simulink library "m3_common_lib"  (R2021b)
settings: Solver=ode45  StartTime=0.0  StopTime=10.0  RelTol=1e-3
undefined symbols (not defined in the file or in its folder): ACCEL_PRE_MULT, APDT_SrvcMgr_IRVHVDCSubFcnReq, C_C1GearNumbers, C_C1GearRatios, C_Calibration, C_DitherWaveform, C_GearOffset, C_GearRatioIn, C_GearRatioInverseOut, C_GearRatioOut, CLUTCH_INNER_LOOP_UPDATE_RATE, CONSTANT, DEGRADED_MODE_SIZE, Dem_EventStatusType, DiscIntNeverNeededParam, F_FAULT_ENUM, F_NOFAULT, F_OUTOFRANGE, F_RATELIMIT, FALSE, FMI14_SPECIAL_INSTRUCTIONS, FMI20_DATA_DRIFTED_HIGH, FMI21_DATA_DRIFTED_LOW, FMI29_RESERVED_FOR_SAE_ASSIGNMENT, FMI30_RESERVED_FOR_SAE_ASSIGNMENT, FMI31_CONDITION_EXISTS, FMI32_NO_FAULT, IC, k_accel, k_mean, MAX_UINT32, MEAN_PRE_MULT, NTriggers, QLTY_SIGNAL_FAILED, QLTY_SIGNAL_FULLY_FUNCTION, QLTY_SIGNAL_SUBSTITUTED_BY_1ST_CHOICE, QLTY_SIGNAL_SUBSTITUTED_BY_2ND_CHOICE, QLTY_SIGNAL_SUBSTITUTED_BY_3RD_CHOICE, QLTY_SIGNAL_SUBSTITUTED_BY_4TH_CHOICE, SAMPLE_TIME_100us, simin, T_TestPoint, TF_FALSE, TF_TRUE, TimeStep, TRUE, WORKSPACE_UPDATE_RATE, Zero, ZERO
libraries: $bdroot x121, simulink x23, simulink_extras x4, MBD_EPS_Local_Blockset x4
(part 6 of 10)

== system m3_common_lib/Diagnostics/OOR Fault Detect Enum ==
  note: Common Library::Diagnostics::Out of Range Fault Detection with Enable for Enum
  in : Inport
  Enable : Inport  Port=2
  Logical Operator1 : Logic  Operator=NOT  AllPortsSameDT=off
  Switch : Switch  Criteria=u2 ~= 0
  detect fault : Subsystem
  false : Constant  Value=false  OutDataTypeStr=boolean
  out : Outport  VectorParamsAs1DForOutWhenUnconnected=off
  fault? : Outport  Port=2  VectorParamsAs1DForOutWhenUnconnected=off
  wires:
  Enable/1 -> detect fault/Enable, Logical Operator1/1
  Switch/1 -> fault?/1
  false/1 -> Switch/1
  detect fault/1(fault set) -> Switch/3
  in/1 -> detect fault/1(In1), out/1
  Logical Operator1/1 -> Switch/2

== system m3_common_lib/Diagnostics/OOR Fault Detection ==
  note: Common Library::Diagnostics::Out of Range Fault Detection with Enable
  in : Inport
  Enable : Inport  Port=2
  Logical Operator1 : Logic  Operator=OR  AllPortsSameDT=off
  Logical Operator2 : Logic  Operator=NOT  AllPortsSameDT=off
  Logical Operator3 : Logic  Operator=NOT  AllPortsSameDT=off
  Logical Operator4 : Logic  Operator=NOT  AllPortsSameDT=off
  Switch : Switch  Criteria=u2 ~= 0
  applyLimits : Constant  Value=applyLimits
  detect fault : Subsystem
  false : Constant  Value=false  OutDataTypeStr=boolean
  out : Outport  VectorParamsAs1DForOutWhenUnconnected=off
  fault? : Outport  Port=2  VectorParamsAs1DForOutWhenUnconnected=off
  wires:
  Enable/1 -> Logical Operator3/1
  in/1 -> out/1, detect fault/1(In1)
  applyLimits/1 -> Logical Operator2/1
  Logical Operator1/1 -> Switch/2, Logical Operator4/1
  detect fault/1(fault set) -> Switch/3
  false/1 -> Switch/1
  Switch/1 -> fault?/1
  Logical Operator2/1 -> Logical Operator1/1
  Logical Operator3/1 -> Logical Operator1/2
  Logical Operator4/1 -> detect fault/Enable

== system m3_common_lib/Diagnostics/SetFMI ==
  FMI_in : Inport  OutDataTypeStr=uint8  PortDimensions=1
  Active1 : Inport  Port=2  OutDataTypeStr=boolean  PortDimensions=1
  Active2 : Inport  Port=3  OutDataTypeStr=boolean  PortDimensions=1
  Active3 : Inport  Port=4  OutDataTypeStr=boolean  PortDimensions=1
  Active4 : Inport  Port=5  OutDataTypeStr=boolean  PortDimensions=1
  Active5 : Inport  Port=6  OutDataTypeStr=boolean  PortDimensions=1
  Active6 : Inport  Port=7  OutDataTypeStr=boolean  PortDimensions=1
  Active7 : Inport  Port=8  OutDataTypeStr=boolean  PortDimensions=1
  Constant : Constant  Value=PRIORITY_1_FMI
  Constant1 : Constant  Value=PRIORITY_2_FMI
  Constant2 : Constant  Value=PRIORITY_3_FMI
  Constant3 : Constant  Value=PRIORITY_4_FMI
  Constant4 : Constant  Value=PRIORITY_5_FMI
  Constant5 : Constant  Value=PRIORITY_6_FMI
  Constant6 : Constant  Value=PRIORITY_7_FMI
  IF_ELSE_LADDER : Subsystem  TreatAsAtomicUnit=on
      settings: RTWSystemCode=Inline
  FMI_out : Outport  VectorParamsAs1DForOutWhenUnconnected=off
  wires:
  IF_ELSE_LADDER/1(FMI_out) -> FMI_out/1
  Active7/1 -> IF_ELSE_LADDER/8(Active7)
  Active6/1 -> IF_ELSE_LADDER/7(Active6)
  Active5/1 -> IF_ELSE_LADDER/6(Active5)
  Active4/1 -> IF_ELSE_LADDER/5(Active4)
  Active3/1 -> IF_ELSE_LADDER/4(Active3)
  Active2/1 -> IF_ELSE_LADDER/3(Active2)
  Active1/1 -> IF_ELSE_LADDER/2(Active1)
  FMI_in/1 -> IF_ELSE_LADDER/1(FMI_in)
  Constant6/1 -> IF_ELSE_LADDER/15(FMI_7)
  Constant5/1 -> IF_ELSE_LADDER/14(FMI_6)
  Constant4/1 -> IF_ELSE_LADDER/13(FMI_5)
  Constant3/1 -> IF_ELSE_LADDER/12(FMI_4)
  Constant2/1 -> IF_ELSE_LADDER/11(FMI_3)
  Constant1/1 -> IF_ELSE_LADDER/10(FMI_2)
  Constant/1 -> IF_ELSE_LADDER/9(FMI_1)

== system m3_common_lib/Diagnostics/SignalSubstitution ==
  Signal_in : Inport  OutDataTypeStr=single  PortDimensions=1
  SignalFaulted : Inport  Port=2  OutDataTypeStr=boolean  PortDimensions=1
  FirstChoiceSubstitute : Inport  Port=3  OutDataTypeStr=single  PortDimensions=1
  FirstChoiceFaulted : Inport  Port=4  OutDataTypeStr=boolean  PortDimensions=1
  SecondChoiceSubstitute : Inport  Port=5  OutDataTypeStr=single  PortDimensions=1
  SecondChoiceFaulted : Inport  Port=6  OutDataTypeStr=boolean  PortDimensions=1
  ThirdChoiceSubstitute : Inport  Port=7  OutDataTypeStr=single  PortDimensions=1
  ThirdChoiceFaulted : Inport  Port=8  OutDataTypeStr=boolean  PortDimensions=1
  FourthChoiceSubstitute : Inport  Port=9  OutDataTypeStr=single  PortDimensions=1
  FourthChoiceFaulted : Inport  Port=10  OutDataTypeStr=boolean  PortDimensions=1
  FailedValue : Inport  Port=11  OutDataTypeStr=single  PortDimensions=1
  If : If  NumInputs=5  IfExpression=~u1  ElseIfExpressions=~u2, ~u3, ~u4, ~u5
  If Action Subsystem : Subsystem  TreatAsAtomicUnit=on
  If Action Subsystem1 : Subsystem  TreatAsAtomicUnit=on
  If Action Subsystem2 : Subsystem  TreatAsAtomicUnit=on
  If Action Subsystem3 : Subsystem  TreatAsAtomicUnit=on
  If Action Subsystem4 : Subsystem  TreatAsAtomicUnit=on
  If Action Subsystem5 : Subsystem  TreatAsAtomicUnit=on
  Merge : Merge  Inputs=6
  Merge1 : Merge  Inputs=6
  Signal_out : Outport  OutDataTypeStr=single  PortDimensions=1  VectorParamsAs1DForOutWhenUnconnected=off
  Qlty : Outport  Port=2  OutDataTypeStr=uint8  PortDimensions=1  VectorParamsAs1DForOutWhenUnconnected=off
  wires:
  If Action Subsystem2/2(Qlty) -> Merge1/3
  If Action Subsystem2/1(Signal) -> Merge/3
  If Action Subsystem1/2(Qlty) -> Merge1/2
  If Action Subsystem3/1(Signal) -> Merge/4
  Merge/1 -> Signal_out/1
  If Action Subsystem4/2(Qlty) -> Merge1/5
  If Action Subsystem/1(Signal) -> Merge/1
  If Action Subsystem4/1(Signal) -> Merge/5
  If Action Subsystem5/1(Signal) -> Merge/6
  If Action Subsystem1/1(Signal) -> Merge/2
  If Action Subsystem3/2(Qlty) -> Merge1/4
  If Action Subsystem/2(Qlty) -> Merge1/1
  If Action Subsystem5/2(Qlty) -> Merge1/6
  Merge1/1 -> Qlty/1
  If/3 -> If Action Subsystem2/Action
  Signal_in/1 -> If Action Subsystem/1(NoSubstitute)
  SecondChoiceSubstitute/1 -> If Action Subsystem2/1(SecondChoice)
  If/1 -> If Action Subsystem/Action
  FirstChoiceFaulted/1 -> If/2
  If/2 -> If Action Subsystem1/Action
  SecondChoiceFaulted/1 -> If/3
  FourthChoiceFaulted/1 -> If/5
  FirstChoiceSubstitute/1 -> If Action Subsystem1/1(FirstChoice)
  If/4 -> If Action Subsystem3/Action
  ThirdChoiceFaulted/1 -> If/4
  FailedValue/1 -> If Action Subsystem5/1(FailedValue)
  If/5 -> If Action Subsystem4/Action
  If/6 -> If Action Subsystem5/Action
  SignalFaulted/1 -> If/1
  FourthChoiceSubstitute/1 -> If Action Subsystem4/1(FourthChoice)
  ThirdChoiceSubstitute/1 -> If Action Subsystem3/1(ThirdChoice)

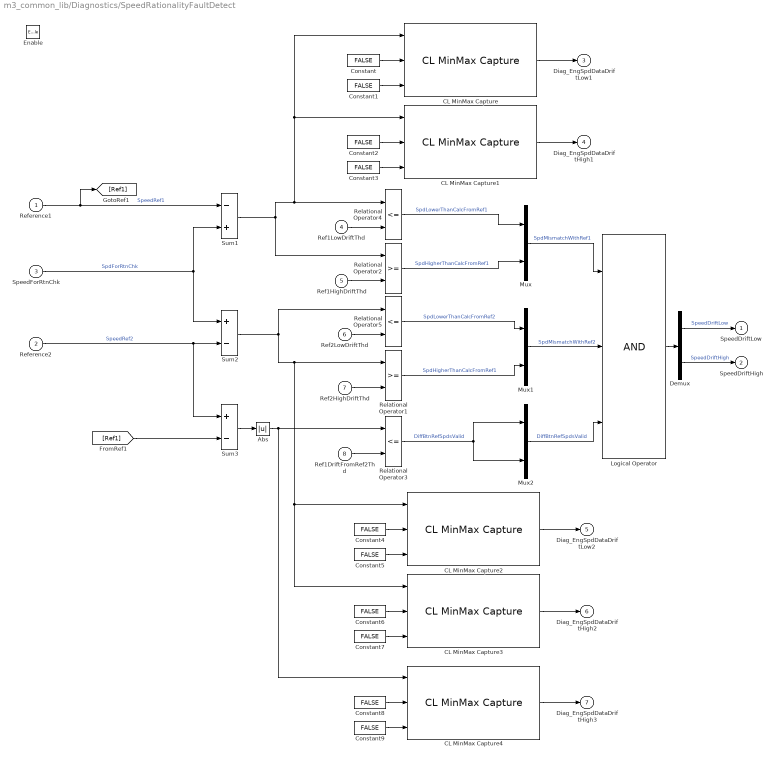
== system m3_common_lib/Diagnostics/SpeedRationalityFaultDetect ==
  Reference1 : Inport
  Reference2 : Inport  Port=2
  SpeedForRtnChk : Inport  Port=3
  Ref1LowDriftThd : Inport  Port=4
  Ref1HighDriftThd : Inport  Port=5
  Ref2LowDriftThd : Inport  Port=6
  Ref2HighDriftThd : Inport  Port=7
  Ref1DriftFromRef2Thd : Inport  Port=8
  Enable : EnablePort  ZeroCross=off
  Abs : Abs  ZeroCross=off
  CL MinMax Capture : $bdroot/Diag/CL MinMax Capture  CaptureType=Min  InDataType=single
  CL MinMax Capture1 : $bdroot/Diag/CL MinMax Capture  CaptureType=Max  InDataType=single
  CL MinMax Capture2 : $bdroot/Diag/CL MinMax Capture  CaptureType=Min  InDataType=single
  CL MinMax Capture3 : $bdroot/Diag/CL MinMax Capture  CaptureType=Max  InDataType=single
  CL MinMax Capture4 : $bdroot/Diag/CL MinMax Capture  CaptureType=Max  InDataType=single
  Constant{,1..9} (10 alike) : Constant  Value=FALSE  SampleTime=-1
  Demux : Demux  Outputs=2
  Logical Operator : Logic  Inputs=3  AllPortsSameDT=off
  Mux : Mux  Inputs=2
  Mux1 : Mux  Inputs=2
  Mux2 : Mux  Inputs=2
  Relational Operator1 : RelationalOperator  ZeroCross=off  RndMeth=Nearest
  Relational Operator2 : RelationalOperator  ZeroCross=off  RndMeth=Nearest
  Relational Operator3 : RelationalOperator  Operator=<=  ZeroCross=off  RndMeth=Nearest
  Relational Operator4 : RelationalOperator  Operator=<=  ZeroCross=off  RndMeth=Nearest
  Relational Operator5 : RelationalOperator  Operator=<=  ZeroCross=off  RndMeth=Nearest
  Sum1 : Sum  Inputs=-+
  Sum2 : Sum  Inputs=+-
  Sum3 : Sum  Inputs=+-
  SpeedDriftLow : Outport  OutputWhenDisabled=reset  InitialOutput=[0]  VectorParamsAs1DForOutWhenUnconnected=off
  SpeedDriftHigh : Outport  Port=2  OutputWhenDisabled=reset  InitialOutput=[0]  VectorParamsAs1DForOutWhenUnconnected=off
  Diag_EngSpdDataDriftLow1 : Outport  Port=3  InitialOutput=[0]  VectorParamsAs1DForOutWhenUnconnected=off
  Diag_EngSpdDataDriftHigh1 : Outport  Port=4  InitialOutput=[0]  VectorParamsAs1DForOutWhenUnconnected=off
  Diag_EngSpdDataDriftLow2 : Outport  Port=5  InitialOutput=[0]  VectorParamsAs1DForOutWhenUnconnected=off
  Diag_EngSpdDataDriftHigh2 : Outport  Port=6  InitialOutput=[0]  VectorParamsAs1DForOutWhenUnconnected=off
  Diag_EngSpdDataDriftHigh3 : Outport  Port=7  InitialOutput=[0]  VectorParamsAs1DForOutWhenUnconnected=off
  wires:
  Constant9/1 -> CL MinMax Capture4/3
  Constant8/1 -> CL MinMax Capture4/2
  CL MinMax Capture4/1 -> Diag_EngSpdDataDriftHigh3/1
  CL MinMax Capture3/1 -> Diag_EngSpdDataDriftHigh2/1
  CL MinMax Capture2/1 -> Diag_EngSpdDataDriftLow2/1
  Constant7/1 -> CL MinMax Capture3/3
  Constant6/1 -> CL MinMax Capture3/2
  Constant5/1 -> CL MinMax Capture2/3
  Constant4/1 -> CL MinMax Capture2/2
  CL MinMax Capture1/1 -> Diag_EngSpdDataDriftHigh1/1
  CL MinMax Capture/1 -> Diag_EngSpdDataDriftLow1/1
  Constant3/1 -> CL MinMax Capture1/3
  Constant2/1 -> CL MinMax Capture1/2
  Constant1/1 -> CL MinMax Capture/3
  Constant/1 -> CL MinMax Capture/2
  Reference2/1 -> Sum3/1, Sum2/2  "SpeedRef2"
  Reference1/1 -> [Ref1], Sum1/1  "SpeedRef1"
  Ref2HighDriftThd/1 -> Relational Operator1/2
  Ref1HighDriftThd/1 -> Relational Operator2/2
  Logical Operator/1 -> Demux/1
  Demux/2 -> SpeedDriftHigh/1  "SpeedDriftHigh"
  Demux/1 -> SpeedDriftLow/1  "SpeedDriftLow"
  Mux2/1 -> Logical Operator/3  "DiffBtnRefSpdsValid"
  Mux1/1 -> Logical Operator/2  "SpdMismatchWithRef2"
  Mux/1 -> Logical Operator/1  "SpdMismatchWithRef1"
  Relational Operator1/1 -> Mux1/2  "SpdHigherThanCalcFromRef1"
  Relational Operator5/1 -> Mux1/1  "SpdLowerThanCalcFromRef2"
  Relational Operator4/1 -> Mux/1  "SpdLowerThanCalcFromRef1"
  Sum3/1 -> Abs/1
  Ref2LowDriftThd/1 -> Relational Operator5/2
  Ref1LowDriftThd/1 -> Relational Operator4/2
  Ref1DriftFromRef2Thd/1 -> Relational Operator3/2
  Abs/1 -> CL MinMax Capture4/1, Relational Operator3/1
  Sum2/1 -> Relational Operator5/1, Relational Operator1/1, CL MinMax Capture3/1, CL MinMax Capture2/1
  [Ref1] -> Sum3/2
  SpeedForRtnChk/1 -> Sum2/1, Sum1/2  "SpdForRtnChk"
  Relational Operator2/1 -> Mux/2  "SpdHigherThanCalcFromRef1"
  Sum1/1 -> Relational Operator2/1, Relational Operator4/1, CL MinMax Capture/1, CL MinMax Capture1/1
  Relational Operator3/1 -> Mux2/2, Mux2/1  "DiffBtnRefSpdsValid"

== system m3_common_lib/Diagnostics/ToRWSignal ==
  in : Inport
  FMI : Inport  Port=2
  Bus Creator2 : BusCreator  Inputs=2  OutDataTypeStr=Bus: BO_InputSignal
  Data Type Conversion1 : DataTypeConversion  OutDataTypeStr=single
  Data Type Conversion2 : DataTypeConversion  OutDataTypeStr=uint8
  out : Outport  VectorParamsAs1DForOutWhenUnconnected=off
  wires:
  FMI/1 -> Data Type Conversion2/1
  Data Type Conversion2/1 -> Bus Creator2/2  "FMI"
  Data Type Conversion1/1 -> Bus Creator2/1  "value"
  in/1 -> Data Type Conversion1/1
  Bus Creator2/1 -> out/1

== system m3_common_lib/Documentation/EatonLogo ==

== system m3_common_lib/Documentation/LegalNoticeEaton ==

== system m3_common_lib/Documentation/RequirementLinks ==
  DocBlock : simulink/Model-Wide Utilities/DocBlock  DocumentType=Text
      content=|
      | REQ_1234

== system m3_common_lib/Documentation/SubsystemPath ==

== system m3_common_lib/Fltrs/Fltr ==
  note: Common Library::Filters::Filter
  input : Inport
  tau : Inport  Port=2
  Constant : Constant  Value=single(0)  SampleTime=-1
  Constant1 : Constant  Value=false  SampleTime=-1
  Constant2 : Constant  Value=false  SampleTime=-1
  Data Type Conversion : DataTypeConversion  OutDataTypeStr=single
  Data Type Conversion1 : DataTypeConversion  OutDataTypeStr=single
  FilterCoreLogic1 : $bdroot/Fltrs/Fltr_wRO/FilterCoreLogic  SystemSampleTime=-1  VariantActivationTime=update diagram  Latency=0  AutoFrameSizeCalculation=off
  Signal Conversion : SignalConversion  ConversionOutput=Contiguous copy  OverrideOpt=on
  output : Outport  VectorParamsAs1DForOutWhenUnconnected=off
  wires:
  input/1 -> Data Type Conversion/1
  tau/1 -> Data Type Conversion1/1
  Signal Conversion/1 -> output/1
  FilterCoreLogic1/1 -> Signal Conversion/1
  Constant/1 -> FilterCoreLogic1/3
  Constant1/1 -> FilterCoreLogic1/4
  Constant2/1 -> FilterCoreLogic1/5
  Data Type Conversion/1 -> FilterCoreLogic1/1
  Data Type Conversion1/1 -> FilterCoreLogic1/2

== system m3_common_lib/Fltrs/Fltr_wR ==
  note: Common Library::Filters::Filter with Reset
  note: This is a simple 1st order filter block with reset.
      |
      |     if reset is true (1) then output=ic
      |    otherwise output = previous output + (input - previous output) * T/tau
  input : Inport
  tau : Inport  Port=2
  ic : Inport  Port=3
  reset? : Inport  Port=4  OutDataTypeStr=boolean
  Constant : Constant  Value=false  SampleTime=-1
  Data Type Conversion : DataTypeConversion  OutDataTypeStr=single
  Data Type Conversion1 : DataTypeConversion  OutDataTypeStr=single
  Data Type Conversion2 : DataTypeConversion  OutDataTypeStr=single
  Data Type Conversion3 : DataTypeConversion  OutDataTypeStr=boolean
  FilterCoreLogic1 : $bdroot/Fltrs/Fltr_wRO/FilterCoreLogic  SystemSampleTime=-1  VariantActivationTime=update diagram  Latency=0  AutoFrameSizeCalculation=off
  Signal Conversion : SignalConversion  ConversionOutput=Contiguous copy  OverrideOpt=on
  output : Outport  VectorParamsAs1DForOutWhenUnconnected=off
  wires:
  ic/1 -> Data Type Conversion2/1
  reset?/1 -> Data Type Conversion3/1
  input/1 -> Data Type Conversion/1
  tau/1 -> Data Type Conversion1/1
  FilterCoreLogic1/1 -> Signal Conversion/1
  Signal Conversion/1 -> output/1
  Constant/1 -> FilterCoreLogic1/5
  Data Type Conversion/1 -> FilterCoreLogic1/1
  Data Type Conversion1/1 -> FilterCoreLogic1/2
  Data Type Conversion2/1 -> FilterCoreLogic1/3
  Data Type Conversion3/1 -> FilterCoreLogic1/4

== system m3_common_lib/Fltrs/Fltr_wRO ==
  note: This is a simple 1st order filter block with reset and override.
      |
      |      If override is true (1) then output=override_value
      |      If       reset is true (1) then output=input
      |    otherwise output = previous output + (input - previous output) * T/tau
  note: Common Library::Filters::Filter with Reset and Override
  input : Inport
  tau : Inport  Port=2
  override_value : Inport  Port=3
  override? : Inport  Port=4  OutDataTypeStr=boolean
  reset? : Inport  Port=5  OutDataTypeStr=boolean
  Data Type Conversion : DataTypeConversion  OutDataTypeStr=single
  Data Type Conversion1 : DataTypeConversion  OutDataTypeStr=single
  Data Type Conversion2 : DataTypeConversion  OutDataTypeStr=single
  Data Type Conversion3 : DataTypeConversion  OutDataTypeStr=boolean
  Data Type Conversion4 : DataTypeConversion  OutDataTypeStr=boolean
  FilterCoreLogic : Subsystem  TreatAsAtomicUnit=on  RTWFcnName=FLTR
      settings: RTWFcnNameOpts=User specified  RTWFileNameOpts=Use function name
  Signal Conversion : SignalConversion  ConversionOutput=Contiguous copy  OverrideOpt=on
  output : Outport  VectorParamsAs1DForOutWhenUnconnected=off
  wires:
  FilterCoreLogic/1(output) -> Signal Conversion/1
  tau/1 -> Data Type Conversion1/1
  input/1 -> Data Type Conversion/1
  Signal Conversion/1 -> output/1
  reset?/1 -> Data Type Conversion4/1
  override_value/1 -> Data Type Conversion2/1
  override?/1 -> Data Type Conversion3/1
  Data Type Conversion/1 -> FilterCoreLogic/1(input)
  Data Type Conversion1/1 -> FilterCoreLogic/2(tau)
  Data Type Conversion2/1 -> FilterCoreLogic/3(override_value)
  Data Type Conversion3/1 -> FilterCoreLogic/4(override?)
  Data Type Conversion4/1 -> FilterCoreLogic/5(reset?)

== system m3_common_lib/Fltrs/Fltr_wROExtInitCond ==
  note: This is a simple 1st order filter block with reset and override.
      |
      |      If override is true (1) then output=override_value
      |      If       reset is true (1) then output=input
      |    otherwise output = previous output + (input - previous output) * T/tau
  note: Common Library::Filters::Filter with Reset and Override
  input : Inport
  tau : Inport  Port=2
  init_cond : Inport  Port=3  OutDataTypeStr=single
  reset : Inport  Port=4  OutDataTypeStr=boolean
  override : Inport  Port=5  OutDataTypeStr=boolean
  override_value : Inport  Port=6
  Constant1 : Constant  Value=Ts
  Data Type Conversion{,1..2,5..6} (5 alike) : DataTypeConversion  OutDataTypeStr=single
  Data Type Conversion3 : DataTypeConversion  OutDataTypeStr=boolean
  Data Type Conversion4 : DataTypeConversion  OutDataTypeStr=boolean
  FilterCoreLogic : Subsystem  RTWFcnName=FLTR
      settings: RTWFcnNameOpts=User specified  RTWFileNameOpts=Use function name
  Signal Conversion : SignalConversion  ConversionOutput=Contiguous copy  OverrideOpt=on
  output : Outport  VectorParamsAs1DForOutWhenUnconnected=off
  wires:
  init_cond/1 -> Data Type Conversion6/1
  FilterCoreLogic/1(output) -> Signal Conversion/1
  tau/1 -> Data Type Conversion1/1
  input/1 -> Data Type Conversion/1
  Signal Conversion/1 -> output/1
  reset/1 -> Data Type Conversion4/1
  override_value/1 -> Data Type Conversion2/1
  override/1 -> Data Type Conversion3/1
  Data Type Conversion3/1 -> FilterCoreLogic/6(override)
  Data Type Conversion2/1 -> FilterCoreLogic/7(override_value)
  Data Type Conversion/1 -> FilterCoreLogic/1(input)
  Data Type Conversion4/1 -> FilterCoreLogic/5(reset)
  Data Type Conversion1/1 -> FilterCoreLogic/2(tau)
  Data Type Conversion6/1 -> FilterCoreLogic/3(init_cond)
  Constant1/1 -> Data Type Conversion5/1
  Data Type Conversion5/1 -> FilterCoreLogic/4(task_rate)

== system m3_common_lib/Fltrs/Int16FIR ==
  u : Inport  OutDataTypeStr=int16
  Accum : Subsystem  TreatAsAtomicUnit=on
  Buffer : simulink/Discrete/Tapped Delay  vinit=0.0  samptime=-1  NumDelays=2*N  DelayOrder=Newest  includeCurrent=off
  Constant : Constant  Value=MEAN_PRE_MULT
  Constant1 : Constant  Value=ACCEL_PRE_MULT
  Constant2 : Constant  Value=int32(N)
  Constant3 : Constant  Value=int32(2^(k_accel-1))
  Constant4 : Constant  Value=int32(2^(k_mean-1))
  Data Type Conversion : DataTypeConversion  OutDataTypeStr=int16  SaturateOnIntegerOverflow=on
  Data Type Conversion1 : DataTypeConversion  OutDataTypeStr=int16
  Data Type Conversion2 : DataTypeConversion  OutDataTypeStr=int32
  Data Type Conversion3 : DataTypeConversion  OutDataTypeStr=int32
  Data Type Conversion4 : DataTypeConversion  OutDataTypeStr=int32
  Product : Product  OutDataTypeStr=int32
  Product1 : Product  OutDataTypeStr=int32
  Product2 : Product  OutDataTypeStr=int32
  Selector : Selector  IndexMode=Zero-based  InputPortWidth=2*N  IndexOptions=Index vector (dialog)  Indices=N-1  OutputSizes=1
  Selector1 : Selector  IndexMode=Zero-based  InputPortWidth=2*N  IndexOptions=Index vector (dialog)  Indices=2*N-1  OutputSizes=1
  Shift Arithmetic : ArithShift  BitShiftNumber=k_mean
  Shift Arithmetic1 : ArithShift  BitShiftNumber=k_accel
  Sum{,1,4..6} (5 alike) : Sum  Inputs=|++
  Sum2 : Sum  Inputs=++|
  Sum3 : Sum  Inputs=|+-
  Mean : Outport  VectorParamsAs1DForOutWhenUnconnected=off
  Accel : Outport  Port=2  VectorParamsAs1DForOutWhenUnconnected=off
  wires:
  Constant4/1 -> Sum6/2
  Sum6/1 -> Shift Arithmetic/1
  Constant3/1 -> Sum5/2
  Sum5/1 -> Shift Arithmetic1/1
  Product2/1 -> Sum4/2
  Sum4/1 -> Product1/1
  Constant2/1 -> Product2/2
  Sum3/1 -> Product2/1
  Data Type Conversion4/1 -> Sum2/1, Sum3/1
  Sum2/1 -> Sum1/2
  Data Type Conversion3/1 -> Sum2/2, Sum3/2
  Data Type Conversion2/1 -> Sum1/1
  Selector1/1 -> Data Type Conversion3/1
  u/1 -> Buffer/1, Data Type Conversion4/1
  Data Type Conversion/1 -> Accel/1
  Sum/1 -> Product/1
  Product/1 -> Sum6/1
  Constant/1 -> Product/2
  Shift Arithmetic/1 -> Data Type Conversion1/1
  Constant1/1 -> Product1/2
  Product1/1 -> Sum5/1
  Buffer/1 -> Accum/1(Buf), Selector/1, Selector1/1
  Shift Arithmetic1/1 -> Data Type Conversion/1
  Accum/1(Accel_Accum) -> Sum4/1
  Selector/1 -> Data Type Conversion2/1
  Data Type Conversion1/1 -> Mean/1
  Sum1/1 -> Sum/2
  Accum/2(Mean_Accum) -> Sum/1

== system m3_common_lib/Fltrs/Inv_Fltr ==
  note: This is the inverse of a simple 1st order filter block
  note: Common Library::Filters::Inverse Filter
  input : Inport
  tau : Inport  Port=2
  Constant1 : Constant  Value=TimeStep
  Constant2 : Constant  Value=false
  Data Type Conversion : DataTypeConversion  OutDataTypeStr=single
  Product : Product  Inputs=*/  InputSameDT=on  OutDataTypeStr=Inherit: Same as first input
  Product1 : Product  Inputs=**  InputSameDT=on  OutDataTypeStr=Inherit: Same as first input
  Sum : Sum  Inputs=-+|  InputSameDT=on  OutDataTypeStr=Inherit: Same as first input
  Sum1 : Sum  Inputs=++|  InputSameDT=on  OutDataTypeStr=Inherit: Same as first input
  Switch1 : Switch  Threshold=0.5  ZeroCross=off  InputSameDT=on
  Unit Delay1 : UnitDelay  InitialCondition=Zero  SampleTime=-1  HasFrameUpgradeWarning=on
      settings: AttributesFormatString=ic=%<X0>
  Unit Delay2 : UnitDelay  InitialCondition=true  SampleTime=-1  HasFrameUpgradeWarning=on
      settings: AttributesFormatString=ic=%<X0>
  output : Outport  VectorParamsAs1DForOutWhenUnconnected=off
  wires:
  Constant1/1 -> Data Type Conversion/1
  Data Type Conversion/1 -> Product/2
  Unit Delay2/1 -> Switch1/2
  Constant2/1 -> Unit Delay2/1
  Switch1/1 -> Sum1/1, Sum/1
  Unit Delay1/1 -> Switch1/3
  Sum1/1 -> output/1
  Product1/1 -> Sum1/2
  Product/1 -> Product1/2
  Sum/1 -> Product1/1
  tau/1 -> Product/1
  input/1 -> Unit Delay1/1, Switch1/1, Sum/2

== system m3_common_lib/Fltrs/Inv_RpdFltr ==
  note: u(k) = y(k-1) + ( y(k) - y(k-1) )/fc
  note: Common Library::Filters::Inverse Rapid Filtering
  input : Inport
  fltr_cnst : Inport  Port=2
  Constant1 : Constant  Value=single(eps)
  Constant3 : Constant  Value=false
  MinMax : MinMax  Function=max  Inputs=2  InputSameDT=on  SaturateOnIntegerOverflow=on  ZeroCross=off
  Product : Product  Inputs=*/  InputSameDT=on  OutDataTypeStr=Inherit: Same as first input
  Sum : Sum  Inputs=|+-  InputSameDT=on  OutDataTypeStr=Inherit: Same as first input
  Sum1 : Sum  Inputs=|++  InputSameDT=on  OutDataTypeStr=Inherit: Same as first input
  Switch2 : Switch  Threshold=0.5  ZeroCross=off  InputSameDT=on
  Unit Delay3 : UnitDelay  InitialCondition=Zero  SampleTime=-1  HasFrameUpgradeWarning=on
      settings: AttributesFormatString=ic=%<X0>
  Unit Delay4 : UnitDelay  InitialCondition=true  SampleTime=-1  HasFrameUpgradeWarning=on
      settings: AttributesFormatString=ic=%<X0>
  output : Outport  VectorParamsAs1DForOutWhenUnconnected=off
  wires:
  Switch2/1 -> Sum/2
  Unit Delay4/1 -> Switch2/2
  Constant3/1 -> Unit Delay4/1
  Unit Delay3/1 -> Switch2/3
  fltr_cnst/1 -> MinMax/2
  MinMax/1 -> Product/2
  Constant1/1 -> MinMax/1
  input/1 -> Switch2/1, Unit Delay3/1, Sum/1
  Sum/1 -> Product/1
  Product/1 -> Sum1/1
  Sum1/1 -> output/1

== system m3_common_lib/Fltrs/Lookup_wFltr ==
  input : Inport
  x-axis_vector : Inport  Port=2
  y-axis_vector : Inport  Port=3
  override? : Inport  Port=4
  override_value : Inport  Port=5
  filter_enable? : Inport  Port=6
  tau : Inport  Port=7
  ic : Inport  Port=8
  2D Lookup : $bdroot/Tbl/2D Lookup
  Fltr_wROExtInitCond : $bdroot/Fltrs/Fltr_wROExtInitCond  TimeStep=Ts
  NOT : Logic  Operator=NOT  AllPortsSameDT=off  OutDataTypeStr=boolean
  output : Outport  VectorParamsAs1DForOutWhenUnconnected=off
  wires:
  Fltr_wROExtInitCond/1 -> output/1
  input/1 -> 2D Lookup/1
  y-axis_vector/1 -> 2D Lookup/3
  x-axis_vector/1 -> 2D Lookup/2
  2D Lookup/1 -> Fltr_wROExtInitCond/1
  filter_enable?/1 -> NOT/1
  NOT/1 -> Fltr_wROExtInitCond/4
  tau/1 -> Fltr_wROExtInitCond/2
  ic/1 -> Fltr_wROExtInitCond/3
  override?/1 -> Fltr_wROExtInitCond/5
  override_value/1 -> Fltr_wROExtInitCond/6

== system m3_common_lib/Fltrs/Rpd_Fltr ==
  note: Common Library::Filters::Rapid Filter
  note: Y(k) = FC * ( X(k) - Y(k-1)) + Y(k-1)
  input : Inport
  fltr_cnst : Inport  Port=2
  Product : Product  Inputs=**  InputSameDT=on  OutDataTypeStr=Inherit: Same as first input
  Sum : Sum  Inputs=|+-  InputSameDT=on  OutDataTypeStr=Inherit: Same as first input
  Sum1 : Sum  Inputs=|++  InputSameDT=on  OutDataTypeStr=Inherit: Same as first input
  Unit Delay : UnitDelay  InitialCondition=IC  SampleTime=-1  HasFrameUpgradeWarning=on
  output : Outport  VectorParamsAs1DForOutWhenUnconnected=off
  wires:
  Sum/1 -> Product/1
  input/1 -> Sum/1
  Unit Delay/1 -> Sum/2, Sum1/2
  fltr_cnst/1 -> Product/2
  Product/1 -> Sum1/1
  Sum1/1 -> output/1, Unit Delay/1

== system m3_common_lib/Fltrs/Scaling_wFltr ==
  input : Inport
  res : Inport  Port=2
  offset : Inport  Port=3
  override : Inport  Port=4
  override_value : Inport  Port=5
  filter_enable : Inport  Port=6
  tau : Inport  Port=7
  init_cond : Inport  Port=8
  Add : Sum
  Fltr_wROExtInitCond : $bdroot/Fltrs/Fltr_wROExtInitCond  TimeStep=Ts
  NOT : Logic  Operator=NOT  AllPortsSameDT=off  OutDataTypeStr=boolean
  Product : Product
  output : Outport  VectorParamsAs1DForOutWhenUnconnected=off
  wires:
  Fltr_wROExtInitCond/1 -> output/1
  res/1 -> Product/2
  Add/1 -> Fltr_wROExtInitCond/1
  offset/1 -> Add/2
  input/1 -> Product/1
  Product/1 -> Add/1
  NOT/1 -> Fltr_wROExtInitCond/4
  filter_enable/1 -> NOT/1
  tau/1 -> Fltr_wROExtInitCond/2
  init_cond/1 -> Fltr_wROExtInitCond/3
  override/1 -> Fltr_wROExtInitCond/5
  override_value/1 -> Fltr_wROExtInitCond/6

== system m3_common_lib/Fuzzy/Fuzzy Implication ==
  THEN : Inport
  Product : Product  RndMeth=Zero
  Select : BusSelector  OutputSignals=HighUpshiftPoint  OutputAsBus=on
  OUTPUT : Outport  VectorParamsAs1DForOutWhenUnconnected=off
  wires:
  THEN/1 -> Product/1
  [ShiftPoint] -> Select/1
  Select/1 -> Product/2
  Product/1 -> OUTPUT/1

== system m3_common_lib/Fuzzy/Fuzzy Intersection ==
  IF : Inport
  MinMax : MinMax  Inputs=2
  OR : Sum  Inputs=+
  Select : BusSelector  OutputSignals=Demand.value
  Sum : Sum  Inputs=|+-
  THEN : Outport  VectorParamsAs1DForOutWhenUnconnected=off
  ELSE : Outport  Port=2  VectorParamsAs1DForOutWhenUnconnected=off
  wires:
  [DataBus] -> Select/1
  OR/1 -> MinMax/2
  MinMax/1 -> Sum/2, THEN/1
  Sum/1 -> ELSE/1
  IF/1 -> Sum/1, MinMax/1
  Select/1 -> OR/1  "<value>"

== system m3_common_lib/Fuzzy/Fuzzy Membership Function ==
  note: Triangle Membership Function
  note: This switch is initializing
      | a vector of zeros equal in
      | length to the breakpoints.
  u : Inport
  brkpts : Inport  Port=2
  Assignment : Assignment  IndexMode=Zero-based  IndexOptions=Index vector (port)  Indices=1  OutputSizes=1
  Assignment1 : Assignment  IndexMode=Zero-based  IndexOptions=Index vector (port)  Indices=1  OutputSizes=1
  Constant2 : Constant  Value=single(0)
  Constant3 : Constant  Value=single(1)
  Constant5 : Constant  Value=true
  Constant6 : Constant  Value=uint32(1)
  Prelookup : PreLookup  BreakpointsDataSource=Input port  BreakpointsData=[10:10:110]  FractionDataTypeStr=single
      settings: InputPortMap=u0,p1
  Sum : Sum  Inputs=|+-
  Sum1 : Sum  Inputs=|++
  Switch : Switch  Threshold=0.5  InputSameDT=on
  Outport : Outport  VectorParamsAs1DForOutWhenUnconnected=off
  wires:
  Constant6/1 -> Sum1/2
  u/1 -> Prelookup/1
  Assignment1/1 -> Outport/1
  brkpts/1 -> Prelookup/2, Switch/3
  Constant5/1 -> Switch/2
  Constant2/1 -> Switch/1
  Switch/1 -> Assignment/1
  Constant3/1 -> Sum/1
  Prelookup/1 -> Sum1/1, Assignment/3
  Sum1/1 -> Assignment1/3
  Assignment/1 -> Assignment1/1
  Sum/1 -> Assignment/2
  Prelookup/2 -> Sum/2, Assignment1/2

== system m3_common_lib/Gear Ratios/FindGearNumberByRatio ==
  note: If either the output speed, or the clutch speed is above minimum
      | then report that the speed is above minimum speed for detection.  However,
      | only output a gear other than zero to the GearNumber if OS > min speed.  This is done
      | because if the OS is stopped, but the clutch speed is still > min, you can tell
      | that there is no ratio being imposed.  So GearNumber should report zero, and the speeds are
      | above the threshold for detecting this condition.
  note: This block finds the gear number that corresponds to the ratio
      | between the os and clutch speed.  The output speed must be above the MinSpeed, and the ratio must be
      | within the SpeedTolerance for at least a time of ConfirmTime before OutputValid goes true.
      | If OutputValid is false then the GearNumber output does not have any meaning.
  OutputSpeed : Inport
  ClutchSpeed : Inport  Port=2
  SpeedTolerance : Inport  Port=3
  MinSpeed : Inport  Port=4
  Abs : Abs  ZeroCross=off
  Abs1 : Abs  ZeroCross=off
  Abs2 : Abs  ZeroCross=off
  ClampAroundZero : $bdroot/Misc/ClampAroundZero  Tol=single(0.1)
      settings: AttributesFormatString=tol=%<Tol>
  Constant1 : Constant  Value=ConfirmTime
  Constant2 : Constant  Value=single(0)
  GearToRatio : Lookup  InputValues=GearToRatioIn  Table=GearToRatioOut  LookUpMeth=Use Input Nearest
  Logical Operator : Logic  AllPortsSameDT=off
  Logical Operator1 : Logic  Operator=OR  AllPortsSameDT=off
  Product1 : Product  Inputs=/*  RndMeth=Zero
  Product2 : Product  Inputs=**  RndMeth=Zero
  RatioToGear : Lookup  InputValues=RatioToGearIn  Table=RatioToGearOut  LookUpMeth=Use Input Nearest
  Relational Operator : RelationalOperator  Operator=<  ZeroCross=off  RndMeth=Nearest
  Relational Operator1 : RelationalOperator  Operator=>  ZeroCross=off  RndMeth=Nearest
  Relational Operator2 : RelationalOperator  Operator=>  ZeroCross=off  RndMeth=Nearest
  Sum : Sum  Inputs=-+
  Switch : Switch  Threshold=0.5  ZeroCross=off
  Timer1 : Subsystem  mask{TimeStep=0}
      mask prompts: TimeStep "Time Step (double)"
      mask help:
      | This block outputs a boolean true when In has been true
      | for at least the TiggerTime time.
  GearNumber : Outport  VectorParamsAs1DForOutWhenUnconnected=off
  OutputValid : Outport  Port=2  VectorParamsAs1DForOutWhenUnconnected=off
  SpeedAboveMin : Outport  Port=3  VectorParamsAs1DForOutWhenUnconnected=off
  wires:
  Relational Operator2/1 -> Logical Operator1/2
  Abs2/1 -> Relational Operator2/1
  Logical Operator1/1 -> SpeedAboveMin/1
  ClampAroundZero/1 -> Product1/1, Product2/2, Abs1/1
  Constant1/1 -> Timer1/2(TriggerTime)
  Timer1/1(Out) -> Switch/2, OutputValid/1
  Logical Operator/1 -> Timer1/1(In)
  Product1/1 -> RatioToGear/1
  ClutchSpeed/1 -> Abs2/1, Sum/2, Product1/2
  RatioToGear/1 -> GearToRatio/1, Switch/1  "nearest_gear_number"
  GearToRatio/1 -> Product2/1  "nearest_ratio"
  Product2/1 -> Sum/1  "nearest_speed_byratio"
  Abs/1 -> Relational Operator/1
  Sum/1 -> Abs/1
  SpeedTolerance/1 -> Relational Operator/2
  Relational Operator/1 -> Logical Operator/1
  Constant2/1 -> Switch/3
  OutputSpeed/1 -> ClampAroundZero/1
  Switch/1 -> GearNumber/1
  Abs1/1 -> Relational Operator1/1
  MinSpeed/1 -> Relational Operator2/2, Relational Operator1/2
  Relational Operator1/1 -> Logical Operator1/1, Logical Operator/2

== system m3_common_lib/Gear Ratios/GearNumberToRatio ==
  gear_number : Inport
  C_GearInverseRatio : LookupNDDirect  NumberOfTableDimensions=1  Table=C_GearRatioInverseOut
  C_GearRatio : LookupNDDirect  NumberOfTableDimensions=1  Table=C_GearRatioOut
  Constant5 : Constant  Value=int8(-99)  SampleTime=-1
  GearOffset : Constant  Value=C_GearOffset  SampleTime=-1
  GearOffset1 : Constant  Value=int8(0)  SampleTime=-1
  Relational Operator3 : RelationalOperator  Operator=~=  ZeroCross=off  RndMeth=Nearest  InputSameDT=on
  Subtract : Sum
  Switch : Switch  Threshold=0.5  ZeroCross=off
  ratio : Outport  VectorParamsAs1DForOutWhenUnconnected=off
  inv_ratio : Outport  Port=2  VectorParamsAs1DForOutWhenUnconnected=off
  wires:
  GearOffset1/1 -> Switch/3
  Relational Operator3/1 -> Switch/2
  Constant5/1 -> Relational Operator3/2
  GearOffset/1 -> Subtract/2
  Subtract/1 -> C_GearRatio/1, C_GearInverseRatio/1
  Switch/1 -> Subtract/1
  gear_number/1 -> Switch/1, Relational Operator3/1
  C_GearRatio/1 -> ratio/1
  C_GearInverseRatio/1 -> inv_ratio/1

== system m3_common_lib/IO/Calibration with Pretty Print Value ==
  C_Calibration : Constant  Value=CalValue  SampleTime=-1
  Outport : Outport  VectorParamsAs1DForOutWhenUnconnected=off
  wires:
  C_Calibration/1 -> Outport/1

== system m3_common_lib/IO/From Workspace w//Datatype ==
  Data Type Conversion : DataTypeConversion
  From Workspace : FromWorkspace  VariableName=var  SampleTime=st  ZeroCross=off
  Out1 : Outport  VectorParamsAs1DForOutWhenUnconnected=off
  wires:
  From Workspace/1 -> Data Type Conversion/1
  Data Type Conversion/1 -> Out1/1

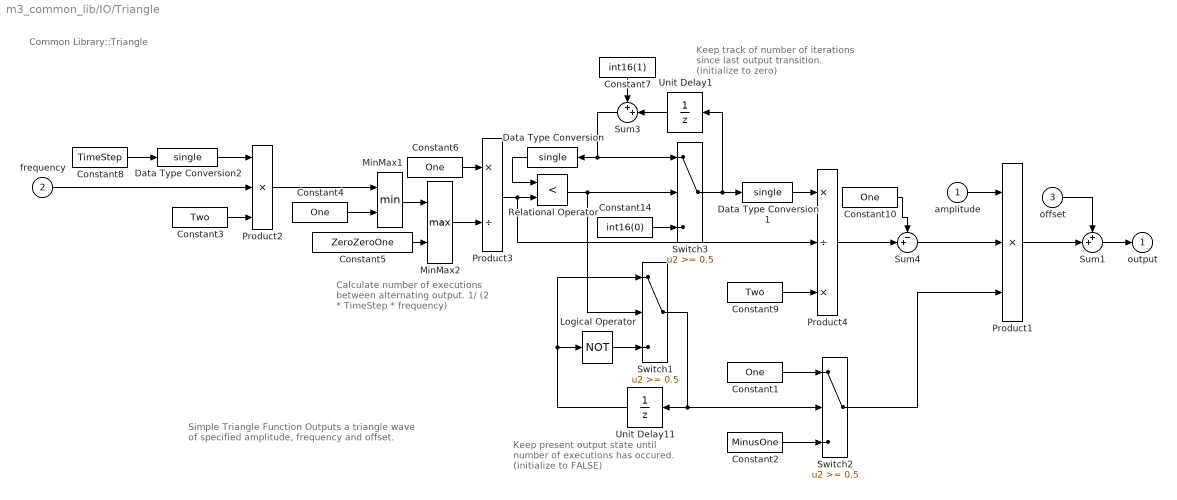
== system m3_common_lib/IO/Triangle ==
  note: Common Library::Triangle
  note: Simple Triangle Function
      | Outputs a triangle wave of specified
      | amplitude, frequency and offset.
  note: Calculate number of executions
      | between alternating output.
      | 1/ (2 * TimeStep * frequency)
  note: Keep track of number of iterations
      | since last output transition.
      | (initialize to zero)
  note: Keep present output state until
      | number of executions has occured.
      | (initialize to FALSE)
  amplitude : Inport
  frequency : Inport  Port=2
  offset : Inport  Port=3
  Constant{1,4,6,10} (4 alike) : Constant  Value=One
  Constant14 : Constant  Value=int16(0)
  Constant2 : Constant  Value=MinusOne
  Constant3 : Constant  Value=Two
  Constant5 : Constant  Value=ZeroZeroOne
  Constant7 : Constant  Value=int16(1)
  Constant8 : Constant  Value=TimeStep
  Constant9 : Constant  Value=Two
  Data Type Conversion : DataTypeConversion  OutDataTypeStr=single  RndMeth=Zero
  Data Type Conversion1 : DataTypeConversion  OutDataTypeStr=single  RndMeth=Zero
  Data Type Conversion2 : DataTypeConversion  OutDataTypeStr=single
  Logical Operator : Logic  Operator=NOT
  MinMax1 : MinMax  Inputs=2  InputSameDT=on  SaturateOnIntegerOverflow=on  ZeroCross=off
  MinMax2 : MinMax  Function=max  Inputs=2  InputSameDT=on  SaturateOnIntegerOverflow=on  ZeroCross=off
  Product1 : Product  Inputs=3  InputSameDT=on  OutDataTypeStr=Inherit: Same as first input
  Product2 : Product  Inputs=***  InputSameDT=on  OutDataTypeStr=Inherit: Same as first input
  Product3 : Product  Inputs=*/  InputSameDT=on  OutDataTypeStr=Inherit: Same as first input
  Product4 : Product  Inputs=*/*  InputSameDT=on  OutDataTypeStr=Inherit: Same as first input
  Relational Operator : RelationalOperator  Operator=<  ZeroCross=off  RndMeth=Nearest  InputSameDT=on
  Sum1 : Sum  Inputs=++|  InputSameDT=on  OutDataTypeStr=Inherit: Same as first input
  Sum3 : Sum  Inputs=++|  InputSameDT=on  OutDataTypeStr=Inherit: Same as first input
  Sum4 : Sum  Inputs=-+|  InputSameDT=on  OutDataTypeStr=Inherit: Same as first input
  Switch1 : Switch  Threshold=0.5  ZeroCross=off  InputSameDT=on
  Switch2 : Switch  Threshold=0.5  ZeroCross=off  InputSameDT=on
  Switch3 : Switch  Threshold=0.5  ZeroCross=off  InputSameDT=on
  Unit Delay1 : UnitDelay  SampleTime=-1  HasFrameUpgradeWarning=on
  Unit Delay11 : UnitDelay  InitialCondition=false  SampleTime=-1  HasFrameUpgradeWarning=on
  output : Outport  VectorParamsAs1DForOutWhenUnconnected=off
  wires:
  Constant8/1 -> Data Type Conversion2/1
  Data Type Conversion2/1 -> Product2/1
  Switch2/1 -> Product1/3
  Constant2/1 -> Switch2/3
  Constant1/1 -> Switch2/1
  Sum4/1 -> Product1/2
  Product4/1 -> Sum4/2
  Constant10/1 -> Sum4/1
  Constant9/1 -> Product4/3
  Data Type Conversion1/1 -> Product4/1
  offset/1 -> Sum1/1
  Unit Delay11/1 -> Logical Operator/1, Switch1/1
  Switch1/1 -> Switch2/2, Unit Delay11/1
  Product1/1 -> Sum1/2
  amplitude/1 -> Product1/1
  frequency/1 -> Product2/2
  Product2/1 -> MinMax1/1
  Constant4/1 -> MinMax1/2
  MinMax1/1 -> MinMax2/1
  Constant5/1 -> MinMax2/2
  Sum1/1 -> output/1
  MinMax2/1 -> Product3/2
  Constant6/1 -> Product3/1
  Constant3/1 -> Product2/3
  Switch3/1 -> Data Type Conversion1/1, Unit Delay1/1
  Constant14/1 -> Switch3/3
  Unit Delay1/1 -> Sum3/2
  Constant7/1 -> Sum3/1
  Sum3/1 -> Switch3/1, Data Type Conversion/1
  Logical Operator/1 -> Switch1/3
  Product3/1 -> Product4/2, Relational Operator/2
  Relational Operator/1 -> Switch3/2, Switch1/2
  Data Type Conversion/1 -> Relational Operator/1

== system m3_common_lib/Integrators/ForwardEulerIntergrator ==
  dx : Inport
  x0 : Inport  Port=2
  reset : Inport  Port=3
  Constant2 : Constant  Value=TSAMP  SampleTime=-1
  Data Type Conversion : DataTypeConversion  OutDataTypeStr=single  RndMeth=Zero
  Divide : Product  Inputs=**
  Sum : Sum  Inputs=|++
  Switch1 : Switch  Threshold=0.5  ZeroCross=off
  Unit Delay : UnitDelay  InitialCondition=IC  SampleTime=-1  HasFrameUpgradeWarning=on
      settings: AttributesFormatString=ic=%<X0>
  x : Outport  VectorParamsAs1DForOutWhenUnconnected=off
  wires:
  Data Type Conversion/1 -> Divide/2
  Sum/1 -> Unit Delay/1
  Unit Delay/1 -> Switch1/3
  Switch1/1 -> x/1, Sum/2
  x0/1 -> Switch1/1
  reset/1 -> Switch1/2
  dx/1 -> Divide/1
  Divide/1 -> Sum/1
  Constant2/1 -> Data Type Conversion/1

== system m3_common_lib/Misc/ArcSine ==
  note: Common Library::Trigonometry:Sine
  note: Taylor Series Expansion for ArcSIN
      | Best Accuracy from -pi/3 to +pi/3
  angle : Inport
  Constant5 : Constant  Value=single(1/6)
  Constant6 : Constant  Value=single(3/40)
  Constant7 : Constant  Value=single(15/336)
  Constant9 : Constant  Value=single(105/3456)
  Product{1..2,4..5} (4 alike) : Product  OutDataTypeStr=Inherit: Same as first input
  Product{3,6..8} (4 alike) : Product  Inputs=3  OutDataTypeStr=Inherit: Same as first input
  Sum1 : Sum  Inputs=5
  asin : Outport  VectorParamsAs1DForOutWhenUnconnected=off
  wires:
  Sum1/1 -> asin/1
  Product6/1 -> Product4/1
  Product4/1 -> Sum1/5
  angle/1 -> Product7/2, Sum1/1, Product8/1, Product8/2, Product8/3, Product7/3, Product3/2, Product3/3, Product6/3, Product6/2
  Constant9/1 -> Product4/2
  Product2/1 -> Sum1/4
  Constant7/1 -> Product2/2
  Product3/1 -> Product2/1, Product6/1
  Product1/1 -> Sum1/3
  Constant6/1 -> Product1/2
  Product7/1 -> Product1/1, Product3/1
  Product5/1 -> Sum1/2
  Constant5/1 -> Product5/2
  Product8/1 -> Product7/1, Product5/1

== system m3_common_lib/Misc/ClampAboveZero ==
  note: Common Library::Miscellaneous Computations::Clamp Above Zero
  input : Inport
  Constant : Constant  Value=Tol
  MinMax : MinMax  Function=max  Inputs=2  InputSameDT=on  SaturateOnIntegerOverflow=on  ZeroCross=off
  output : Outport  VectorParamsAs1DForOutWhenUnconnected=off
  wires:
  input/1 -> MinMax/1
  MinMax/1 -> output/1
  Constant/1 -> MinMax/2

== system m3_common_lib/Misc/ClampAroundZero ==
  note: Common Library::Miscellaneous Computations::Clamp Around Zero
  input : Inport
  Abs : Abs  ZeroCross=off
  Constant : Constant  Value=Tol
  Constant1 : Constant  Value=Zero
  Constant2 : Constant  Value=One
  Constant3 : Constant  Value=MinusOne
  MinMax : MinMax  Function=max  Inputs=2  InputSameDT=on  SaturateOnIntegerOverflow=on  ZeroCross=off
  Product : Product  InputSameDT=on  OutDataTypeStr=Inherit: Same as first input
  Relational Operator : RelationalOperator  ZeroCross=off  RndMeth=Nearest  InputSameDT=on
  Switch1 : Switch  Threshold=0.5  ZeroCross=off  InputSameDT=on
  output : Outport  VectorParamsAs1DForOutWhenUnconnected=off
  wires:
  Constant/1 -> MinMax/2
  Abs/1 -> MinMax/1
  input/1 -> Abs/1, Relational Operator/1
  MinMax/1 -> Product/2
  Switch1/1 -> Product/1
  Product/1 -> output/1
  Constant1/1 -> Relational Operator/2
  Relational Operator/1 -> Switch1/2
  Constant2/1 -> Switch1/1
  Constant3/1 -> Switch1/3

== system m3_common_lib/Misc/Cosine ==
  note: Taylor Series Expansion for COS(x)
  note: Common Library::Trigonometry:Cosine
  angle : Inport
  Constant : Constant  Value=single(1/(1*2))
  Constant1 : Constant  Value=single(1/(1*2*3*4))
  Constant2 : Constant  Value=single(1)
  Product : Product  OutDataTypeStr=Inherit: Same as first input
  Product1 : Product  OutDataTypeStr=Inherit: Same as first input
  Product3 : Product  OutDataTypeStr=Inherit: Same as first input
  Product6 : Product  Inputs=3  OutDataTypeStr=Inherit: Same as first input
  Sum : Sum  Inputs=+-+
  cos : Outport  VectorParamsAs1DForOutWhenUnconnected=off
  wires:
  Product/1 -> Sum/2
  Product1/1 -> Sum/3
  Sum/1 -> cos/1
  angle/1 -> Product3/2, Product6/2, Product6/3, Product3/1
  Product3/1 -> Product6/1, Product/1
  Constant1/1 -> Product1/2
  Constant/1 -> Product/2
  Product6/1 -> Product1/1
  Constant2/1 -> Sum/1

== system m3_common_lib/Misc/Count Edges ==
  note: Common Library::Miscellaneous::Count Edges
  Input : Inport
  Reset : Inport  Port=2
  Logical Operator5 : Logic  Operator=NOT  AllPortsSameDT=off
  Logical Operator6 : Logic  AllPortsSameDT=off
  Sum : Sum  Inputs=|++  InputSameDT=on  OutDataTypeStr=Inherit: Same as first input
  Switch1 : Switch  Threshold=0.5  ZeroCross=off
  Switch2 : Switch  Threshold=0.5  ZeroCross=off
  Unit Delay2 : UnitDelay  InitialCondition=int8(0)  SampleTime=-1  HasFrameUpgradeWarning=on
      settings: AttributesFormatString=ic=%<X0>
  Unit Delay3 : UnitDelay  InitialCondition=true  SampleTime=-1  HasFrameUpgradeWarning=on
      settings: AttributesFormatString=ic=%<X0>
  constant7 : Constant  Value=int8(0)
  constant8 : Constant  Value=int8(1)
  constant9 : Constant  Value=int8(0)
  Count : Outport  VectorParamsAs1DForOutWhenUnconnected=off
  wires:
  Reset/1 -> Switch1/2
  Input/1 -> Logical Operator6/1, Unit Delay3/1
  Switch1/1 -> Sum/2
  Unit Delay2/1 -> Count/1, Switch1/3
  constant9/1 -> Switch1/1
  Switch2/1 -> Sum/1
  Logical Operator6/1 -> Switch2/2
  Logical Operator5/1 -> Logical Operator6/2
  Unit Delay3/1 -> Logical Operator5/1
  constant8/1 -> Switch2/1
  constant7/1 -> Switch2/3
  Sum/1 -> Unit Delay2/1

== system m3_common_lib/Misc/Count to X ==
  note: Common Library::Miscellaneous::Count to X
  input : Inport
  reset? : Inport  Port=2
  Constant1 : Constant  Value=uint8(1)
  Constant2 : Constant  Value=uint8(0)
  Constant3 : Constant  Value=uint8(X)
  Constant4 : Constant  Value=uint8(0)
  DelayedInput : Logic  Operator=NAND
  Input : Logic
  Logical Operator8 : Logic
  MinMax : MinMax  Inputs=2  InputSameDT=on  SaturateOnIntegerOverflow=on  ZeroCross=off
  Relational Operator : RelationalOperator  ZeroCross=off  RndMeth=Nearest  InputSameDT=on
  Sum1 : Sum  Inputs=++|  InputSameDT=on  OutDataTypeStr=Inherit: Same as first input
  Unit Delay : UnitDelay  InitialCondition=uint8(0)  SampleTime=-1  HasFrameUpgradeWarning=on
  Unit Delay2 : UnitDelay  InitialCondition=false  SampleTime=-1  HasFrameUpgradeWarning=on
  inc switch : Switch  Threshold=0.5  ZeroCross=off  InputSameDT=on
  reset switch : Switch  Threshold=0.5  ZeroCross=off  InputSameDT=on
  output : Outport  VectorParamsAs1DForOutWhenUnconnected=off
  wires:
  Relational Operator/1 -> output/1
  Constant3/1 -> Relational Operator/2, MinMax/1
  Constant2/1 -> inc switch/3
  Constant1/1 -> inc switch/1
  Constant4/1 -> reset switch/1
  input/1 -> Unit Delay2/1, Input/1, Input/2
  Input/1 -> Logical Operator8/1
  Unit Delay2/1 -> DelayedInput/1, DelayedInput/2
  DelayedInput/1 -> Logical Operator8/2
  inc switch/1 -> Sum1/2
  Logical Operator8/1 -> inc switch/2
  Sum1/1 -> Relational Operator/1, MinMax/2
  reset switch/1 -> Sum1/1
  Unit Delay/1 -> reset switch/3
  reset?/1 -> reset switch/2
  MinMax/1 -> Unit Delay/1

== system m3_common_lib/Misc/Counter ==
  note: Counter increments when "incr condition" is TRUE and decrements when "decr condition" is TRUE.
  note: Common Library::Miscellaneous::Counter
  up_val : Inport
  count_up? : Inport  Port=2  OutDataTypeStr=boolean
  down_val : Inport  Port=3
  count_down? : Inport  Port=4  OutDataTypeStr=boolean
  max_count : Inport  Port=5
  min_count : Inport  Port=6
  reset? : Inport  Port=7  OutDataTypeStr=boolean
  Constant1 : Constant  Value=Zero
  Constant2 : Constant  Value=Zero
  Constant4 : Constant  Value=IC
  Constant5 : Constant  Value=false
  Logical Operator : Logic  Operator=OR
  Sat : $bdroot/Slink/Sat
  Sum : Sum  Inputs=++-  InputSameDT=on  OutDataTypeStr=Inherit: Same as first input
  Unit Delay : UnitDelay  InitialCondition=IC  SampleTime=-1  HasFrameUpgradeWarning=on
  Unit Delay1 : UnitDelay  InitialCondition=true  SampleTime=-1  HasFrameUpgradeWarning=on
  dec switch : Switch  Threshold=0.5  ZeroCross=off  InputSameDT=on
  inc switch : Switch  Threshold=0.5  ZeroCross=off  InputSameDT=on
  reset switch : Switch  Threshold=0.5  ZeroCross=off  InputSameDT=on
  output : Outport  VectorParamsAs1DForOutWhenUnconnected=off
  wires:
  count_down?/1 -> dec switch/2
  down_val/1 -> dec switch/1
  count_up?/1 -> inc switch/2
  up_val/1 -> inc switch/1
  Constant2/1 -> dec switch/3
  dec switch/1 -> Sum/3
  Constant1/1 -> inc switch/3
  inc switch/1 -> Sum/2
  reset?/1 -> Logical Operator/1
  reset switch/1 -> Unit Delay/1, output/1
  Unit Delay/1 -> Sum/1
  Logical Operator/1 -> reset switch/2
  Unit Delay1/1 -> Logical Operator/2
  Constant5/1 -> Unit Delay1/1
  Sat/1 -> reset switch/3
  Constant4/1 -> reset switch/1
  max_count/1 -> Sat/2
  min_count/1 -> Sat/3
  Sum/1 -> Sat/1

== system m3_common_lib/Misc/Divide by X ==
  note: Common Library::Miscellaneous::Divide by X
  trigger? : Inport
  Constant1 : Constant  Value=uint8(X)
  Constant2 : Constant  Value=uint8(1)
  Constant3 : Constant  Value=uint8(X)
  Constant4 : Constant  Value=uint8(0)
  Relational Operator : RelationalOperator  ZeroCross=off  RndMeth=Nearest  InputSameDT=on
  Sum1 : Sum  Inputs=|++  InputSameDT=on  OutDataTypeStr=Inherit: Same as first input
  Unit Delay : UnitDelay  InitialCondition=uint8(X)  SampleTime=-1  HasFrameUpgradeWarning=on
  inc switch : Switch  Threshold=0.5  ZeroCross=off  InputSameDT=on
  reset switch : Switch  Threshold=0.5  ZeroCross=off  InputSameDT=on
  output : Outport  VectorParamsAs1DForOutWhenUnconnected=off
  wires:
  Constant4/1 -> reset switch/1
  Constant1/1 -> inc switch/1
  Constant2/1 -> Sum1/1
  trigger?/1 -> inc switch/2
  Sum1/1 -> inc switch/3
  inc switch/1 -> Relational Operator/1, reset switch/3
  Constant3/1 -> Relational Operator/2
  Unit Delay/1 -> Sum1/2
  Relational Operator/1 -> reset switch/2, output/1
  reset switch/1 -> Unit Delay/1

== system m3_common_lib/Misc/EatonLogo ==

== system m3_common_lib/Misc/EdgeTriggered Pulse ==
  note: Common Library::Miscellaneous::Edge Triggered Pulse
  input : Inport
  ETP : $bdroot/Misc/EdgeTriggered Pulse w time  Edge=TRUE to FALSE  Pulse=TRUE  TimeStep=[]  Init=0
  Timeout Threshold : Constant  Value=Width
  pulse : Outport  VectorParamsAs1DForOutWhenUnconnected=off
  wires:
  input/1 -> ETP/1
  Timeout Threshold/1 -> ETP/2
  ETP/1 -> pulse/1

== system m3_common_lib/Misc/EdgeTriggered Pulse w time ==
  note: 0 = PULSE_FALSE
      | 1 = PULSE_TRUE
  note: 0 = FALSE_TO_TRUE
      | 1 = TRUE_TO_FALSE
  input : Inport  OutDataTypeStr=boolean
  width : Inport  Port=2  OutDataTypeStr=single
  Data Type Conversion : DataTypeConversion  OutDataTypeStr=single
  EdgeTriggeredPulseCoreLogic : Subsystem  TreatAsAtomicUnit=on  RTWFcnName=ETPWT
      settings: RTWSystemCode=Inline  RTWFcnNameOpts=User specified  RTWFileNameOpts=Use function name
  Output : Constant  Value=OUTPUT
  Trigger : Constant  Value=TRIGGER
  XOR_IN : Logic  Operator=XOR
  XOR_OUT : Logic  Operator=XOR
  pulse : Outport  OutDataTypeStr=boolean  VectorParamsAs1DForOutWhenUnconnected=off
  wires:
  XOR_IN/1 -> EdgeTriggeredPulseCoreLogic/1(input)
  width/1 -> Data Type Conversion/1
  Output/1 -> XOR_OUT/1
  EdgeTriggeredPulseCoreLogic/1(pulse) -> XOR_OUT/2
  XOR_OUT/1 -> pulse/1
  input/1 -> XOR_IN/2
  Trigger/1 -> XOR_IN/1
  Data Type Conversion/1 -> EdgeTriggeredPulseCoreLogic/2(width)

== system m3_common_lib/Misc/GreenLeaf_Globe ==

== system m3_common_lib/Misc/Hold ==
  in : Inport
  Enable : EnablePort  ZeroCross=off
  out : Outport  VectorParamsAs1DForOutWhenUnconnected=off
  wires:
  in/1 -> out/1

== system m3_common_lib/Misc/Latch ==
  note: Output signal is latched to true until reset input is true.
  note: Common Library::Miscellaneous::Latch
  input : Inport  OutDataTypeStr=boolean
  reset? : Inport  Port=2  OutDataTypeStr=boolean
  Constant2 : Constant  Value=false
  Constant3 : Constant  Value=true
  Switch : Switch  Threshold=0.5  ZeroCross=off  InputSameDT=on
  Switch1 : Switch  Threshold=0.5  ZeroCross=off  InputSameDT=on
  Unit Delay1 : UnitDelay  InitialCondition=IC  SampleTime=-1  HasFrameUpgradeWarning=on
  output : Outport  VectorParamsAs1DForOutWhenUnconnected=off
  wires:
  Switch/1 -> Unit Delay1/1, output/1
  reset?/1 -> Switch/2
  Constant2/1 -> Switch/1
  Switch1/1 -> Switch/3
  Unit Delay1/1 -> Switch1/3
  input/1 -> Switch1/2
  Constant3/1 -> Switch1/1
